simulink library "usask_hyd_lib_simulink"  (R2017a)
settings: Solver=ode45  StartTime=0.0  StopTime=10.0  RelTol=1e-3
undefined symbols (not defined in the file or in its folder): Cd, d, L, magnitude, nu, Re_cr, rho
undefined symbols (not defined in the file): A_l, A_TAmax, P_crTA, P_orTA
libraries: usask_hyd_lib_simulink x1
settings Model: Creator=tkw954  LastModifiedBy=tkw954
settings DataIOCC: LimitDataPoints=on  SaveFormat=Array  SignalLoggingSaveFormat=ModelDataLogs
settings OptimizationCC: BlockReduction=off  BooleanDataType=off  LifeSpan=inf
settings DebuggingCC: SaveWithParameterizedLinksMsg=none  UnderspecifiedInitializationDetection=Classic  MergeDetectMultiDrivingBlocksExec=none  SignalResolutionControl=TryResolveAllWithWarning  MultiTaskDSMMsg=warning  MultiTaskCondExecSysMsg=none  StateNameClashWarn=warning  StrictBusMsg=None  SFUnexpectedBacktrackingDiag=warning  SFNoUnconditionalDefaultTransitionDiag=warning  SFExecutionAtInitializationDiag=none
settings HardwareCC: ProdBitPerPointer=32  ProdBitPerSizeT=32  ProdBitPerPtrDiffT=32  ProdLargestAtomicFloat=None  ProdIntDivRoundTo=Undefined  ProdEndianess=Unspecified  ProdWordSize=32  ProdHWDeviceType=32-bit Generic  TargetUnknown=on
settings ModelReferenceCC: PropagateSignalLabelsOutOfModel=off
settings GRTTargetCC: TargetLangStandard=C89/C90 (ANSI)  GeneratePreprocessorConditionals=Disable all
settings ConfigComp: CovMetricSettings=dw  CovHtmlReporting=on  CovSaveCumulativeToWorkspaceVar=on  CovSaveSingleToWorkspaceVar=on  CovExternalEMLEnable=off

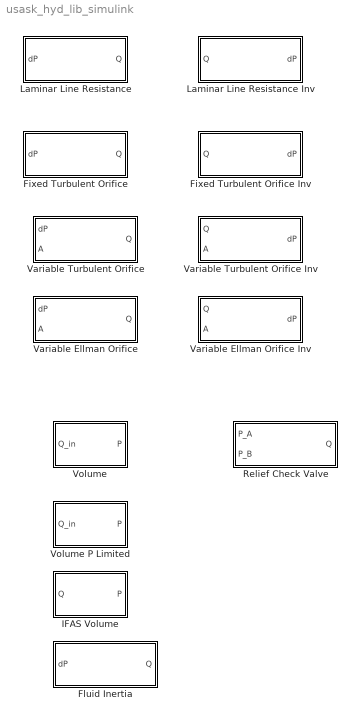
== system usask_hyd_lib_simulink ==
  Fixed Turbulent Orifice : Subsystem  mask(Turbulent Orifice){rho=800, Cd=0.61, A=1e-6}
      mask prompts: rho "Fluid Density (kg/m^3)"; Cd "Discharge Coefficient"; A "Orifice Area (m^2)"
      mask help: This block implements a turbulent orifice equation, with constant area and discharge coefficient.
  Fixed Turbulent Orifice Inv : Subsystem  mask(Turbulent Orifice){rho=800, Cd=0.61, A=1e-6}
      mask prompts: rho "Fluid Density (kg/m^3)"; Cd "Discharge Coefficient"; A "Orifice Area (m^2)"
      mask help: This block implements a turbulent orifice equation, with constant area and discharge coefficient.
  Fluid Inertia : Subsystem  mask(Fluid Inertia){d=d, rho=rho, L=L, Q0=0}
      mask prompts: d "Pipe Diameter (m)"; rho "Fluid Density (kg/m^3)"; L "Pipe Length (m)"; Q0 "Initial Flow (m^3/s)"
      mask help: Implements a simple fluid inertia model for a circular pipe.
  IFAS Volume : Subsystem  mask(Compressible Volume){V=1e-3, P0=101e3, E0=1.55e9, m=11.4, alpha=0.1e-2, Pbeta0=101e3, k=1.4}
      mask prompts: V "Volume (m^3)"; P0 "Initial Pressure (Pa)"; E0 "Oil bulk modulus at zero pressure E0 (Pa)"; m "Oil bulk modulus pressure coefficienct m (Pa/Pa)"; alpha "Entrained air volume fraction at P0"; Pbeta0 "Reference pressure P0 (Pa)"; k "Polytropic constant for air"
      mask help: Implements a compressible volume with variable bulk modulus and contant volume. Uses the IFAS model for pressure-dependent bulk modulus. Pressure is absolute.
  Laminar Line Resistance : Subsystem  mask(Turbulent Orifice){L=1, d=0.012, mu=100e-3}
      mask prompts: L "Length (m)"; d "diameter (m)"; mu "Dynamic Viscosity (Pa s)"
      mask help: This block implements a Hagen Poiseuille pipe flow model. This is for laminar flow through circular pipes.
  Laminar Line Resistance Inv : Subsystem  mask(Turbulent Orifice){L=1, d=0.012, mu=100e-3}
      mask prompts: L "Length (m)"; d "diameter (m)"; mu "Dynamic Viscosity (Pa s)"
      mask help: This block implements a Hagen Poiseuille pipe flow model. This is for laminar flow through circular pipes.
  Relief Check Valve : Subsystem  mask(Static Relief/Check Valve){P_cr=P_crTA, dP_or=P_orTA, A_max=A_TAmax, Cd=Cd, rho=rho, nu=nu, Re_cr=9.3, A_l=1e-9}
      mask prompts: P_cr "Cracking Pressure (Pa)"; dP_or "Pressure Override (Pa)"; A_max "Max Orifice Area (m^2)"; Cd "Discharge Coefficient"; rho "Fluid Density (kg/m^3)"; nu "Fluid Kinematic Viscosity (m^2/s)"; Re_cr "Critical Reynolds Number"; A_l "Leakage Area (m^2)"
      mask help: Implements a static relief or check valve. Valve begins to open at the cracking pressure and continues to open over the pressure override range.
  Variable Ellman Orifice : Subsystem  mask(Turbulent Orifice){rho=800, nu=30e-6, Cd=0.61, Re_cr=12, A0=1e-9}
      mask prompts: rho "Fluid Density (kg/m^3)"; nu "Fluid Kinematic Viscosity (m^2/s)"; Cd "Discharge Coefficient"; Re_cr "Critical Reynolds Number"; A0 "Lekage Area (m^2)"
      mask help: This block implements Ellman's two region orifice equation. This implementation calculates hydraulic diameter assuming a circular orifice.
  Variable Ellman Orifice Inv : Subsystem  mask(Turbulent Orifice){rho=rho, nu=nu, Cd=Cd, Re_cr=Re_cr, A0=A_l}
      mask prompts: rho "Fluid Density (kg/m^3)"; nu "Fluid Kinematic Viscosity (m^2/s)"; Cd "Discharge Coefficient"; Re_cr "Critical Reynolds Number"; A0 "Lekage Area (m^2)"
      mask help: This block implements Ellman's two region orifice equation. This implementation calculates hydraulic diameter assuming a circular orifice.
  Variable Turbulent Orifice : Subsystem  mask(Turbulent Orifice){rho=800, Cd=0.61, A0=1e-9}
      mask prompts: rho "Fluid Density (kg/m^3)"; Cd "Discharge Coefficient"; A0 "Leakage Area (m^2)"
      mask help: This block implements a turbulent orifice equation, with constant discharge coefficient.
  Variable Turbulent Orifice Inv : Subsystem  mask(Turbulent Orifice){rho=800, Cd=0.61, A0=1e-6}
      mask prompts: rho "Fluid Density (kg/m^3)"; Cd "Discharge Coefficient"; A0 "Leakage Area (m^2)"
      mask help: This block implements a turbulent orifice equation, with variable area and constant discharge coefficient.
  Volume : Subsystem  mask(Compressible Volume){V=1e-3, B=1e9, P0=0}
      mask prompts: V "Volume (m^3)"; B "Bulk Modulus (Pa)"; P0 "Initial Pressure (Pa)"
      mask help: Implements a simple compressible volume with constant bulk modulus and volume. No cavitation model is included.
  Volume P Limited : Subsystem  mask(Compressible Volume){V=1e-3, B=1e9, P0=0, P_max=inf, P_min=0}
      mask prompts: V "Volume (m^3)"; B "Bulk Modulus (Pa)"; P0 "Initial Pressure (Pa)"; P_max "Max Pressure (Pa)"; P_min "Min Pressure (Pa)"
      mask help: Implements a simple compressible volume with constant bulk modulus and volume. Minimum and maximum pressures may be specified.

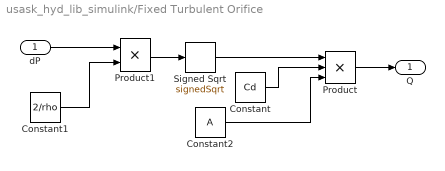
== system usask_hyd_lib_simulink/Fixed Turbulent Orifice ==
  dP : Inport
  Constant : Constant  Value=Cd
  Constant1 : Constant  Value=2/rho
  Constant2 : Constant  Value=A
  Product : Product  Inputs=3
  Product1 : Product
  Signed Sqrt : Sqrt  Operator=signedSqrt  SaturateOnIntegerOverflow=on
  Q : Outport
  wires:
  Constant2/1 -> Product/3
  Constant1/1 -> Product1/2
  dP/1 -> Product1/1
  Product1/1 -> Signed Sqrt/1
  Constant/1 -> Product/2
  Signed Sqrt/1 -> Product/1
  Product/1 -> Q/1

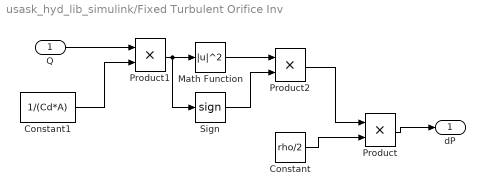
== system usask_hyd_lib_simulink/Fixed Turbulent Orifice Inv ==
  Q : Inport
  Constant : Constant  Value=rho/2
  Constant1 : Constant  Value=1/(Cd*A)
  Math Function : Math  Operator=magnitude^2  SaturateOnIntegerOverflow=on
  Product : Product
  Product1 : Product
  Product2 : Product
  Sign : Signum
  dP : Outport
  wires:
  Product2/1 -> Product/1
  Sign/1 -> Product2/2
  Math Function/1 -> Product2/1
  Q/1 -> Product1/1
  Product/1 -> dP/1
  Constant/1 -> Product/2
  Product1/1 -> Math Function/1, Sign/1
  Constant1/1 -> Product1/2

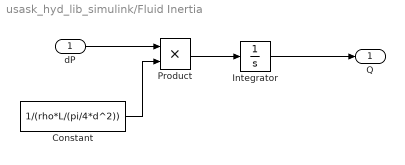
== system usask_hyd_lib_simulink/Fluid Inertia ==
  dP : Inport
  Constant : Constant  Value=1/(rho*L/(pi/4*d^2))
  Integrator : Integrator  InitialCondition=Q0  ZeroCross=off
  Product : Product
  Q : Outport
  wires:
  Product/1 -> Integrator/1
  Constant/1 -> Product/2
  dP/1 -> Product/1
  Integrator/1 -> Q/1

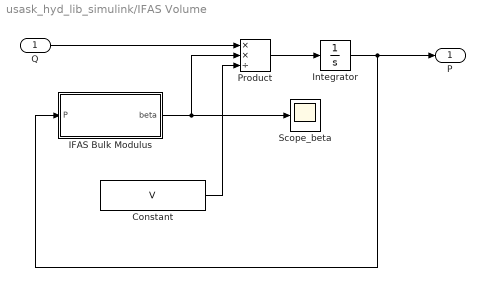
== system usask_hyd_lib_simulink/IFAS Volume ==
  Q : Inport
  Constant : Constant  Value=V
  IFAS Bulk Modulus : Subsystem
  Integrator : Integrator  InitialCondition=P0  ZeroCross=off
  Product : Product  Inputs=**/
  Scope_beta : Scope
  P : Outport
  wires:
  Product/1 -> Integrator/1
  Constant/1 -> Product/3
  Q/1 -> Product/1
  Integrator/1 -> IFAS Bulk Modulus/1(P), P/1
  IFAS Bulk Modulus/1(beta) -> Scope_beta/1, Product/2

== system usask_hyd_lib_simulink/Laminar Line Resistance ==
  dP : Inport
  Constant1 : Constant  Value=pi*d^4/(128*mu*L)
  Product1 : Product
  Q : Outport
  wires:
  Product1/1 -> Q/1
  dP/1 -> Product1/1
  Constant1/1 -> Product1/2

== system usask_hyd_lib_simulink/Laminar Line Resistance Inv ==
  Q : Inport
  Constant1 : Constant  Value=(128*mu*L)/(pi*d^4)
  Product1 : Product
  dP : Outport
  wires:
  Product1/1 -> dP/1
  Q/1 -> Product1/1
  Constant1/1 -> Product1/2

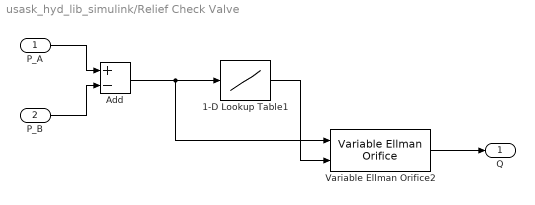
== system usask_hyd_lib_simulink/Relief Check Valve ==
  P_A : Inport
  P_B : Inport  Port=2
  1-D Lookup Table1 : Lookup_n-D  NumberOfTableDimensions=1  BreakpointsForDimension1=[P_cr P_cr+dP_or]  Table=A_max*[0 1]  ExtrapMethod=Clip  InternalRulePriority=Speed  RndMeth=Simplest  InputSameDT=on
  Add : Sum  Inputs=+-
  Variable Ellman Orifice2 : usask_hyd_lib_simulink/Variable Ellman Orifice  rho=rho  nu=nu  Cd=Cd  Re_cr=Re_cr  A0=A_l
      settings: SourceProductName=USask Hydraulic Library Simulink
  Q : Outport
  wires:
  Variable Ellman Orifice2/1 -> Q/1
  P_B/1 -> Add/2
  P_A/1 -> Add/1
  1-D Lookup Table1/1 -> Variable Ellman Orifice2/2
  Add/1 -> 1-D Lookup Table1/1, Variable Ellman Orifice2/1

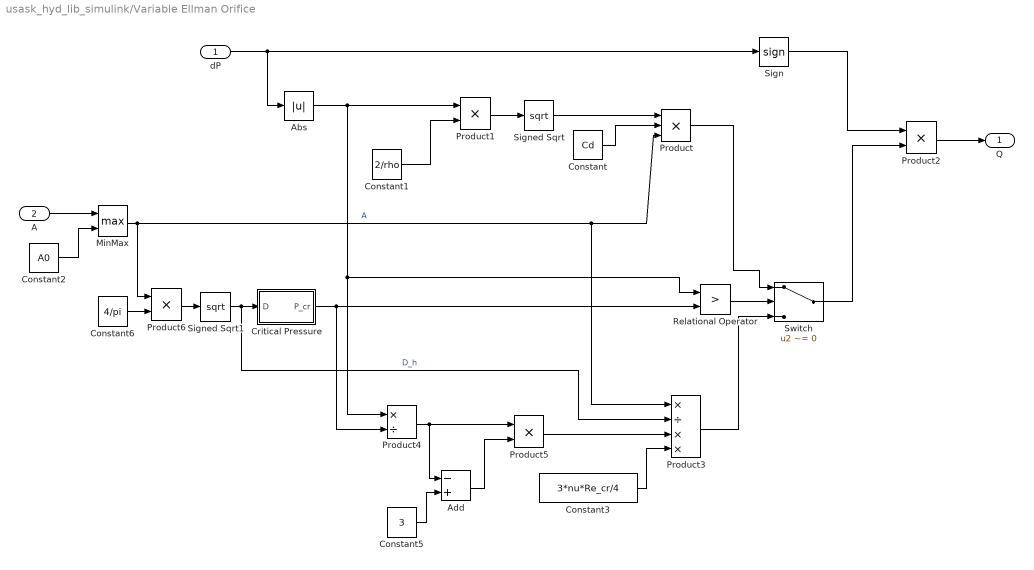
== system usask_hyd_lib_simulink/Variable Ellman Orifice ==
  dP : Inport
  A : Inport  Port=2
  Abs : Abs  ZeroCross=off
  Add : Sum  Inputs=-+
  Constant : Constant  Value=Cd
  Constant1 : Constant  Value=2/rho
  Constant2 : Constant  Value=A0
  Constant3 : Constant  Value=3*nu*Re_cr/4
  Constant5 : Constant  Value=3
  Constant6 : Constant  Value=4/pi
  Critical Pressure : Subsystem
  MinMax : MinMax  Function=max  Inputs=2
  Product : Product  Inputs=3
  Product1 : Product
  Product2 : Product
  Product3 : Product  Inputs=*/**
  Product4 : Product  Inputs=*/
  Product5 : Product  Inputs=**
  Product6 : Product
  Relational Operator : RelationalOperator  Operator=>  OutDataTypeStr=boolean  ZeroCross=off  RndMeth=Nearest
  Sign : Signum  ZeroCross=off
  Signed Sqrt : Sqrt  SaturateOnIntegerOverflow=on
  Signed Sqrt1 : Sqrt  SaturateOnIntegerOverflow=on
  Switch : Switch  Criteria=u2 ~= 0  ZeroCross=off
  Q : Outport
  wires:
  Signed Sqrt/1 -> Product/1
  Constant/1 -> Product/2
  Product1/1 -> Signed Sqrt/1
  dP/1 -> Sign/1, Abs/1
  Constant1/1 -> Product1/2
  A/1 -> MinMax/1
  MinMax/1 -> Product6/1, Product3/1, Product/3  "A"
  Constant2/1 -> MinMax/2
  Product2/1 -> Q/1
  Sign/1 -> Product2/1
  Switch/1 -> Product2/2
  Relational Operator/1 -> Switch/2
  Abs/1 -> Product4/1, Relational Operator/1, Product1/1
  Product/1 -> Switch/1
  Product3/1 -> Switch/3
  Constant3/1 -> Product3/4
  Product5/1 -> Product3/3
  Product4/1 -> Add/1, Product5/1
  Constant5/1 -> Add/2
  Add/1 -> Product5/2
  Product6/1 -> Signed Sqrt1/1
  Signed Sqrt1/1 -> Product3/2, Critical Pressure/1(D)  "D_h"
  Constant6/1 -> Product6/2
  Critical Pressure/1(P_cr) -> Relational Operator/2, Product4/2

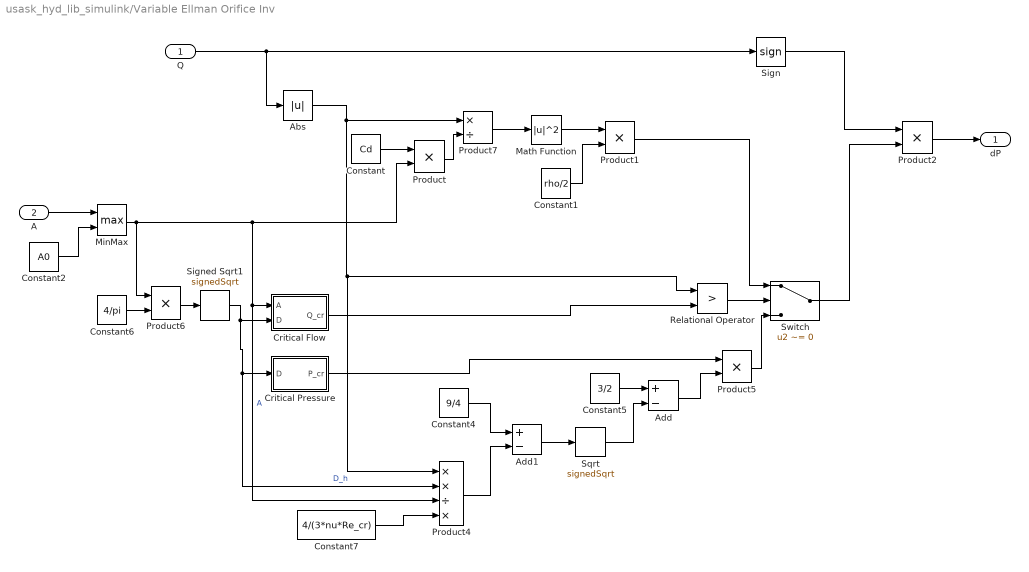
== system usask_hyd_lib_simulink/Variable Ellman Orifice Inv ==
  Q : Inport
  A : Inport  Port=2
  Abs : Abs
  Add : Sum  Inputs=+-
  Add1 : Sum  Inputs=+-
  Constant : Constant  Value=Cd
  Constant1 : Constant  Value=rho/2
  Constant2 : Constant  Value=A0
  Constant4 : Constant  Value=9/4
  Constant5 : Constant  Value=3/2
  Constant6 : Constant  Value=4/pi
  Constant7 : Constant  Value=4/(3*nu*Re_cr)
  Critical Flow : Subsystem
  Critical Pressure : Subsystem
  Math Function : Math  Operator=magnitude^2  SaturateOnIntegerOverflow=on
  MinMax : MinMax  Function=max  Inputs=2
  Product{,1..2,6} (4 alike) : Product
  Product4 : Product  Inputs=**/*
  Product5 : Product  Inputs=**
  Product7 : Product  Inputs=*/
  Relational Operator : RelationalOperator  Operator=>  OutDataTypeStr=boolean  RndMeth=Nearest
  Sign : Signum  ZeroCross=off
  Signed Sqrt1 : Sqrt  Operator=signedSqrt  SaturateOnIntegerOverflow=on
  Sqrt : Sqrt  Operator=signedSqrt  SaturateOnIntegerOverflow=on
  Switch : Switch  Criteria=u2 ~= 0  ZeroCross=off
  dP : Outport
  wires:
  Constant7/1 -> Product4/4
  Product4/1 -> Add1/2
  Constant4/1 -> Add1/1
  Add1/1 -> Sqrt/1
  Sqrt/1 -> Add/2
  Add/1 -> Product5/2
  Critical Pressure/1(P_cr) -> Product5/1
  Math Function/1 -> Product1/1
  Product7/1 -> Math Function/1
  Product/1 -> Product7/2
  Critical Flow/1(Q_cr) -> Relational Operator/2
  Constant6/1 -> Product6/2
  Signed Sqrt1/1 -> Critical Pressure/1(D), Product4/2, Critical Flow/2(D)  "D_h"
  Product6/1 -> Signed Sqrt1/1
  Constant5/1 -> Add/1
  Product5/1 -> Switch/3
  Product1/1 -> Switch/1
  Relational Operator/1 -> Switch/2
  Switch/1 -> Product2/2
  Sign/1 -> Product2/1
  Product2/1 -> dP/1
  Constant2/1 -> MinMax/2
  MinMax/1 -> Product/2, Critical Flow/1(A), Product4/3, Product6/1  "A"
  A/1 -> MinMax/1
  Constant1/1 -> Product1/2
  Q/1 -> Abs/1, Sign/1
  Constant/1 -> Product/1
  Abs/1 -> Relational Operator/1, Product4/1, Product7/1

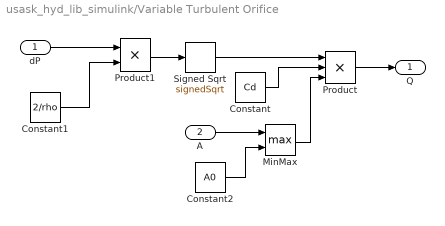
== system usask_hyd_lib_simulink/Variable Turbulent Orifice ==
  dP : Inport
  A : Inport  Port=2
  Constant : Constant  Value=Cd
  Constant1 : Constant  Value=2/rho
  Constant2 : Constant  Value=A0
  MinMax : MinMax  Function=max  Inputs=2
  Product : Product  Inputs=3
  Product1 : Product
  Signed Sqrt : Sqrt  Operator=signedSqrt  SaturateOnIntegerOverflow=on
  Q : Outport
  wires:
  Constant2/1 -> MinMax/2
  MinMax/1 -> Product/3
  A/1 -> MinMax/1
  Constant1/1 -> Product1/2
  dP/1 -> Product1/1
  Product1/1 -> Signed Sqrt/1
  Constant/1 -> Product/2
  Signed Sqrt/1 -> Product/1
  Product/1 -> Q/1

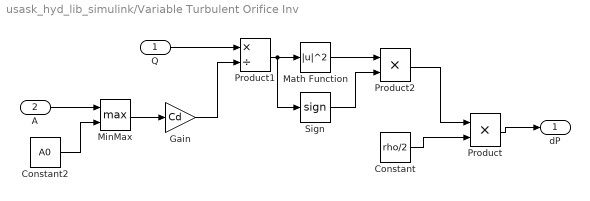
== system usask_hyd_lib_simulink/Variable Turbulent Orifice Inv ==
  Q : Inport
  A : Inport  Port=2
  Constant : Constant  Value=rho/2
  Constant2 : Constant  Value=A0
  Gain : Gain  Gain=Cd
  Math Function : Math  Operator=magnitude^2  SaturateOnIntegerOverflow=on
  MinMax : MinMax  Function=max  Inputs=2
  Product : Product
  Product1 : Product  Inputs=*/
  Product2 : Product
  Sign : Signum
  dP : Outport
  wires:
  Gain/1 -> Product1/2
  MinMax/1 -> Gain/1
  Constant2/1 -> MinMax/2
  A/1 -> MinMax/1
  Product2/1 -> Product/1
  Sign/1 -> Product2/2
  Math Function/1 -> Product2/1
  Q/1 -> Product1/1
  Product/1 -> dP/1
  Constant/1 -> Product/2
  Product1/1 -> Math Function/1, Sign/1

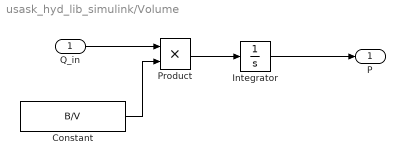
== system usask_hyd_lib_simulink/Volume ==
  Q_in : Inport
  Constant : Constant  Value=B/V
  Integrator : Integrator  InitialCondition=P0  ZeroCross=off
  Product : Product
  P : Outport
  wires:
  Integrator/1 -> P/1
  Q_in/1 -> Product/1
  Constant/1 -> Product/2
  Product/1 -> Integrator/1

== system usask_hyd_lib_simulink/Volume P Limited ==
  Q_in : Inport
  Constant : Constant  Value=B/V
  Integrator : Integrator  InitialCondition=P0  LimitOutput=on  UpperSaturationLimit=P_max  LowerSaturationLimit=P_min
  Product : Product
  P : Outport
  wires:
  Product/1 -> Integrator/1
  Constant/1 -> Product/2
  Q_in/1 -> Product/1
  Integrator/1 -> P/1

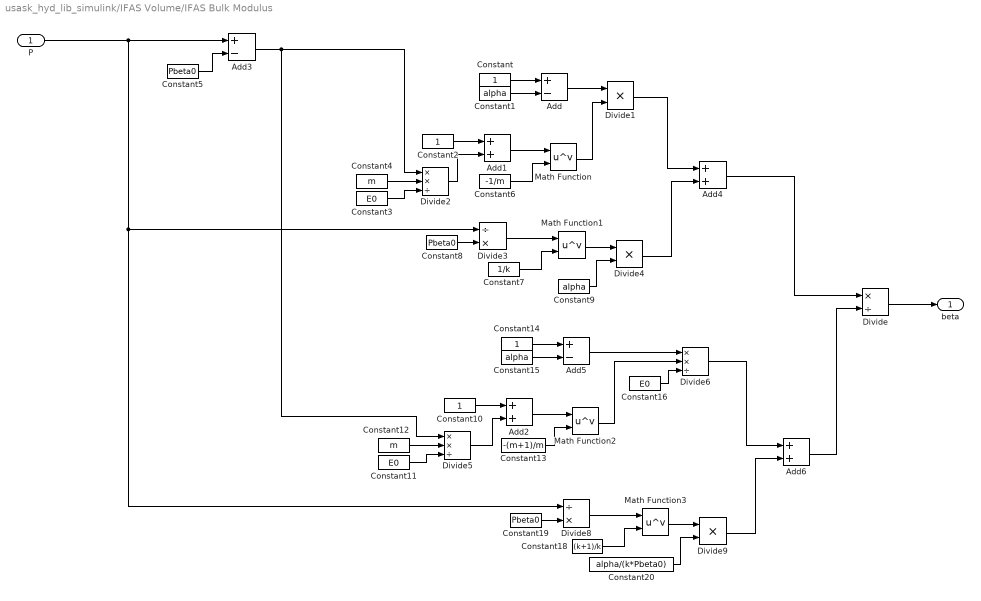
== system usask_hyd_lib_simulink/IFAS Volume/IFAS Bulk Modulus ==
  P : Inport
  Add : Sum  Inputs=+-
  Add{1..2,4,6} (4 alike) : Sum
  Add3 : Sum  Inputs=+-
  Add5 : Sum  Inputs=+-
  Constant{,2,10,14} (4 alike) : Constant
  Constant1 : Constant  Value=alpha
  Constant11 : Constant  Value=E0
  Constant12 : Constant  Value=m
  Constant13 : Constant  Value=-(m+1)/m
  Constant15 : Constant  Value=alpha
  Constant16 : Constant  Value=E0
  Constant18 : Constant  Value=(k+1)/k
  Constant19 : Constant  Value=Pbeta0
  Constant20 : Constant  Value=alpha/(k*Pbeta0)
  Constant3 : Constant  Value=E0
  Constant4 : Constant  Value=m
  Constant5 : Constant  Value=Pbeta0
  Constant6 : Constant  Value=-1/m
  Constant7 : Constant  Value=1/k
  Constant8 : Constant  Value=Pbeta0
  Constant9 : Constant  Value=alpha
  Divide : Product  Inputs=*/
  Divide1 : Product  Inputs=**
  Divide2 : Product  Inputs=**/
  Divide3 : Product  Inputs=/*
  Divide4 : Product  Inputs=**
  Divide5 : Product  Inputs=**/
  Divide6 : Product  Inputs=**/
  Divide8 : Product  Inputs=/*
  Divide9 : Product  Inputs=**
  Math Function{,1..3} (4 alike) : Math  Operator=pow  SaturateOnIntegerOverflow=on
  beta : Outport
  wires:
  Divide/1 -> beta/1
  Constant/1 -> Add/1
  Constant1/1 -> Add/2
  Add/1 -> Divide1/1
  Constant2/1 -> Add1/1
  Divide2/1 -> Add1/2
  Add1/1 -> Math Function/1
  Math Function/1 -> Divide1/2
  Constant6/1 -> Math Function/2
  Constant3/1 -> Divide2/3
  Constant4/1 -> Divide2/2
  Constant5/1 -> Add3/2
  Divide1/1 -> Add4/1
  Constant7/1 -> Math Function1/2
  Divide3/1 -> Math Function1/1
  Constant8/1 -> Divide3/2
  Math Function1/1 -> Divide4/1
  Constant9/1 -> Divide4/2
  Divide4/1 -> Add4/2
  Constant10/1 -> Add2/1
  Divide5/1 -> Add2/2
  Add2/1 -> Math Function2/1
  Constant13/1 -> Math Function2/2
  Constant11/1 -> Divide5/3
  Constant12/1 -> Divide5/2
  Add3/1 -> Divide5/1, Divide2/1
  Constant14/1 -> Add5/1
  Constant15/1 -> Add5/2
  Add5/1 -> Divide6/1
  Math Function2/1 -> Divide6/2
  Constant16/1 -> Divide6/3
  Constant18/1 -> Math Function3/2
  Divide8/1 -> Math Function3/1
  Constant19/1 -> Divide8/2
  Math Function3/1 -> Divide9/1
  Constant20/1 -> Divide9/2
  Divide9/1 -> Add6/2
  Divide6/1 -> Add6/1
  P/1 -> Divide8/1, Divide3/1, Add3/1
  Add4/1 -> Divide/1
  Add6/1 -> Divide/2

== system usask_hyd_lib_simulink/Variable Ellman Orifice/Critical Pressure ==
  D : Inport
  Constant5 : Constant  Value=9*Re_cr^2*rho*nu^2/(8*Cd^2)
  Math Function : Math  Operator=magnitude^2  SaturateOnIntegerOverflow=on
  Product5 : Product  Inputs=*/
  P_cr : Outport
  wires:
  Constant5/1 -> Product5/1
  D/1 -> Math Function/1
  Product5/1 -> P_cr/1
  Math Function/1 -> Product5/2

== system usask_hyd_lib_simulink/Variable Ellman Orifice Inv/Critical Flow ==
  A : Inport
  D : Inport  Port=2
  Constant5 : Constant  Value=3/2*Re_cr*nu
  Product5 : Product  Inputs=**/
  Q_cr : Outport
  wires:
  A/1 -> Product5/2
  D/1 -> Product5/3
  Product5/1 -> Q_cr/1
  Constant5/1 -> Product5/1

== system usask_hyd_lib_simulink/Variable Ellman Orifice Inv/Critical Pressure ==
  D : Inport
  Constant5 : Constant  Value=9*Re_cr^2*rho*nu^2/(8*Cd^2)
  Math Function : Math  Operator=magnitude^2  SaturateOnIntegerOverflow=on
  Product5 : Product  Inputs=*/
  P_cr : Outport
  wires:
  Math Function/1 -> Product5/2
  Product5/1 -> P_cr/1
  D/1 -> Math Function/1
  Constant5/1 -> Product5/1
